simulink model "Working_MBD_UseCases"  (R2025a)
settings: Solver=VariableStepAuto  StartTime=0.0  StopTime=10.0  RelTol=1e-3
libraries: simulink x1
settings Model: Creator=mahij  LastModifiedBy=mahij

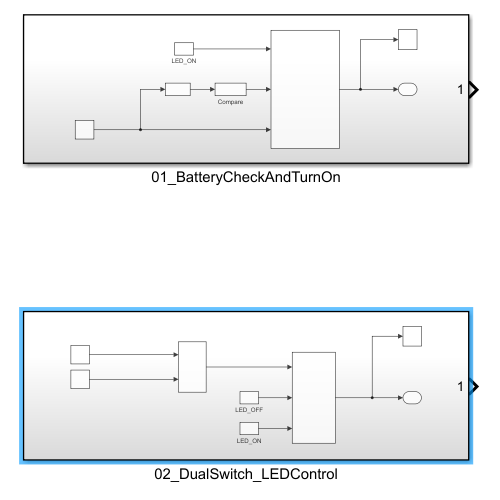
[thumbnail: Simulink's stored preview of the top-level diagram]
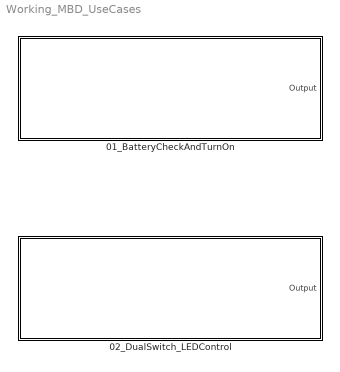
== system Working_MBD_UseCases ==
  01_BatteryCheckAndTurnOn : Subsystem
  02_DualSwitch_LEDControl : Subsystem

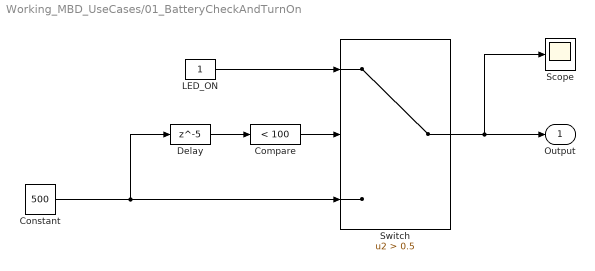
== system Working_MBD_UseCases/01_BatteryCheckAndTurnOn ==
  Compare : simulink/Logic and Bit Operations/Compare To Constant  relop=<  const=100  OutDataTypeStr=boolean
  Constant : Constant  Value=500
  Delay : Delay  DelayLength=5
  LED_ON : Constant
  Scope : Scope
      settings: ActiveDisplayYMinimum=-61.374999999999986  ActiveDisplayYMaximum=562.375
  Switch : Switch  Criteria=u2 > Threshold  Threshold=0.5  SaturateOnIntegerOverflow=off  InputSameDT=off
  Output : Outport
  wires:
  Constant/1 -> Switch/3, Delay/1
  Delay/1 -> Compare/1
  Compare/1 -> Switch/2
  LED_ON/1 -> Switch/1
  Switch/1 -> Scope/1, Output/1

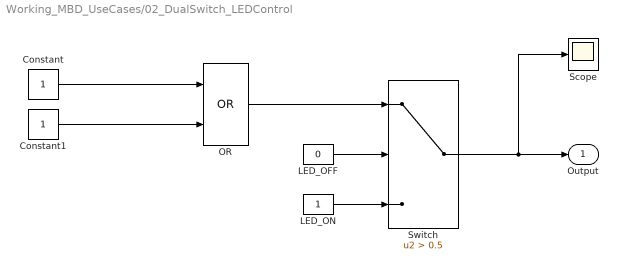
== system Working_MBD_UseCases/02_DualSwitch_LEDControl ==
  Constant : Constant
  Constant1 : Constant
  LED_OFF : Constant  Value=0
  LED_ON : Constant
  OR : Logic  Operator=OR  AllPortsSameDT=off  OutDataTypeStr=boolean
  Scope : Scope
      settings: ActiveDisplayYMinimum=0.9  ActiveDisplayYMaximum=1.1
  Switch : Switch  Criteria=u2 > Threshold  Threshold=0.5  SaturateOnIntegerOverflow=off  InputSameDT=off
  Output : Outport
  wires:
  Constant/1 -> OR/1
  Constant1/1 -> OR/2
  OR/1 -> Switch/1
  LED_OFF/1 -> Switch/2
  LED_ON/1 -> Switch/3
  Switch/1 -> Scope/1, Output/1
